simulink model "FullFilterTest"  (R2019b)
settings: Solver=FixedStepAuto  StartTime=0.0  StopTime=36  FixedStep=1  RelTol=1e-3
libraries: simulink x1
settings Model: Creator=pieterpinson  LastModifiedBy=pieterpinson

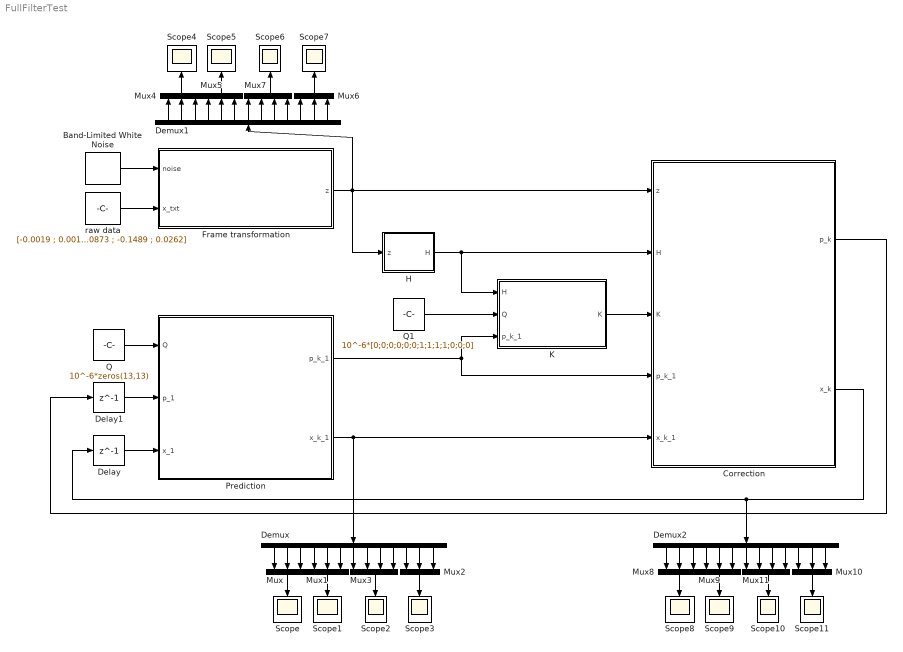
== system FullFilterTest ==
  Band-Limited White Noise : simulink/Sources/Band-Limited White Noise  Cov=[sin(sin(0.1))]  Ts=1  seed=[23341]
  Correction : MATLAB Function  TreatAsAtomicUnit=on
  Delay : Delay  DelayLength=1  InitialCondition=|
      | [-0.0019 ; 0.0017 ; 1.0891 ; 0 ; 0 ; 0 ; -0.7226 ; 0.6358 ; 0.1434 ; 0.2302
      | ; -0.0873 ; -0.1489 ; 0.0262]
  Delay1 : Delay  DelayLength=1  InitialCondition=ones(13,13)
  Demux : Demux  Outputs=13
  Demux1 : Demux  Outputs=13
  Demux2 : Demux  Outputs=13
  Frame transformation : MATLAB Function  TreatAsAtomicUnit=on
  H : MATLAB Function  TreatAsAtomicUnit=on
  K : MATLAB Function  TreatAsAtomicUnit=on
  Mux{,1..2,4..6,8..10} (9 alike) : Mux  Inputs=3
  Mux11 : Mux
  Mux3 : Mux
  Mux7 : Mux
  Prediction : MATLAB Function  TreatAsAtomicUnit=on
  Q : Constant  Value=10^-6*zeros(13,13)
  Q1 : Constant  Value=10^-6*[0;0;0;0;0;0;1;1;1;1;0;0;0]
  Scope{,1..11} (12 alike) : Scope
  raw data : Constant  Value=|
      | [-0.0019 ; 0.0017 ; 1.0891 ; 0 ; 0 ; 0 ; -0.7226 ; 0.6358 ; 0.1434 ; 0.2302
      | ; -0.0873 ; -0.1489 ; 0.0262]
  wires:
  Prediction/2(x_k_1) -> Demux/1, Correction/5(x_k_1)
  Mux3/1 -> Scope2/1
  Demux/13 -> Mux2/3
  Demux/12 -> Mux2/2
  Demux/11 -> Mux2/1
  Demux/10 -> Mux3/4
  Demux/9 -> Mux3/3
  Demux/8 -> Mux3/2
  Demux/7 -> Mux3/1
  Demux/6 -> Mux1/3
  Demux/5 -> Mux1/2
  Demux/4 -> Mux1/1
  Demux/3 -> Mux/3
  Demux/2 -> Mux/2
  Demux/1 -> Mux/1
  Mux1/1 -> Scope1/1
  Mux/1 -> Scope/1
  Delay/1 -> Prediction/3(x_1)
  Mux2/1 -> Scope3/1
  Q/1 -> Prediction/1(Q)
  Delay1/1 -> Prediction/2(p_1)
  raw data/1 -> Frame transformation/2(x_txt)
  Band-Limited White Noise/1 -> Frame transformation/1(noise)
  Mux6/1 -> Scope7/1
  Demux1/3 -> Mux4/3
  Demux1/10 -> Mux7/4
  Demux1/2 -> Mux4/2
  Demux1/1 -> Mux4/1
  Demux1/11 -> Mux6/1
  Mux4/1 -> Scope4/1
  Mux5/1 -> Scope5/1
  Mux7/1 -> Scope6/1
  Demux1/6 -> Mux5/3
  Demux1/9 -> Mux7/3
  Demux1/13 -> Mux6/3
  Demux1/12 -> Mux6/2
  Demux1/7 -> Mux7/1
  Frame transformation/1(z) -> H/1(z), Correction/1(z), Demux1/1
  Demux1/4 -> Mux5/1
  Demux1/5 -> Mux5/2
  Demux1/8 -> Mux7/2
  H/1(H) -> K/1(H), Correction/2(H)
  Correction/1(p_k) -> Delay1/1
  Correction/2(x_k) -> Demux2/1, Delay/1
  Mux10/1 -> Scope11/1
  Demux2/3 -> Mux8/3
  Demux2/10 -> Mux11/4
  Demux2/2 -> Mux8/2
  Demux2/1 -> Mux8/1
  Demux2/11 -> Mux10/1
  Mux8/1 -> Scope8/1
  Mux9/1 -> Scope9/1
  Mux11/1 -> Scope10/1
  Demux2/6 -> Mux9/3
  Demux2/9 -> Mux11/3
  Demux2/4 -> Mux9/1
  Demux2/13 -> Mux10/3
  Demux2/12 -> Mux10/2
  Demux2/7 -> Mux11/1
  Demux2/5 -> Mux9/2
  Demux2/8 -> Mux11/2
  Prediction/1(p_k_1) -> K/3(p_k_1), Correction/4(p_k_1)
  K/1(K) -> Correction/3(K)
  Q1/1 -> K/2(Q)

== matlab function FullFilterTest/Frame transformation ==
  data: noise input; x_txt input; z output
function z = PnPsolver(noise,x_txt)

%PnP solve magie
z = 1*x_txt + noise;

end

== matlab function FullFilterTest/Prediction ==
  data: Q input; p_1 input; p_k_1 output; x_k_1 output; x_1 input
function [p_k_1,x_k_1]= prediction(Q,p_1,x_1)

%orbital parameter
mu = 3.986*10^14;
R_earth = 6371000;
H_target = 773000;
a = R_earth + H_target;
n = sqrt(mu/(a^3));

%clohessy-wiltshire equations
dr = [4-3*cos(n) 0 0 sin(n)/n 2*(1-cos(n))/n 0 ; 6*(sin(n)-n) 1 0 2*(cos(n)-1)/n (4*sin(n)-3*n)/n 0 ; 0 0 cos(n) 0 0 sin(n)/n];
dv = [3*n*sin(n) 0 0 cos(n) 2*sin(n) 0 ; 6*n*(cos(n)-1) 0 0 -2*sin(n) 4*cos(n)-3 0 ; 0 0 -n*sin(n) 0 0 cos(n)];

%quaternion kinematic equation
dq = 0.5*[0 x_1(13) -x_1(12) x_1(11) ; -x_1(13) 0 x_1(11) x_1(12) ; x_1(12) -x_1(11) 0 x_1(13) ; -x_1(11) -x_1(12) -x_1(13) 0];

%state transition matrix
fi = [dr zeros(3,7) ; dv zeros(3,7) ; zeros(4,6) dq zeros(4,3) ; zeros(3,10) eye(3)];

%propogation step
x_k_1 = [0;0;0;0;0;0;x_1(7:10);0;0;0] + fi * x_1;
p_k_1 = fi * p_1 * fi.' + Q;

end


%dq1 = 0.5*[x_1(10) -x_1(9) x_1(8) x_1(7) ; x_1(9) x_1(10) -x_1(7) x_1(8) ; -x_1(8) x_1(7) x_1(10) x_1(9) ; -x_1(7) -x_1(8) -x_1(9) x_1(10)];
%fi(7,7) = x_1(7) + 0.5*(x_1(12)*x_1(8) - x_1(12)*x_1(9) + x_1(11)*x_1(10));
%fi(8,8) = x_1(8) + 0.5*(-x_1(13)*x_1(7) + x_1(11)*x_1(9) + x_1(12)*x_1(10));
%fi(9,9) = x_1(9) + 0.5*(x_1(12)*x_1(7) - x_1(11)*x_1(8) + x_1(13)*x_1(10));
%fi(10,10) = x_1(10) + 0.5*(-x_1(11)*x_1(7) - x_1(12)*x_1(8) - x_1(13)*x_1(9));

== matlab function FullFilterTest/Correction ==
  data: z input; p_k output; x_k output; H input; K input; p_k_1 input; x_k_1 input
function [p_k,x_k]= correction(z,H,K,p_k_1,x_k_1)

%correction step
x_k = x_k_1 + K.*(z - H.'*z);
p_k = (eye(13,13) - K*H)*p_k_1;

end

== matlab function FullFilterTest/H ==
  data: z input; H output
function H = jacobian(z)

%jacobian tranformation magic
H = z;

end

== matlab function FullFilterTest/K ==
  data: H input; Q input; K output; p_k_1 input
function K = kalmangain(H,Q,p_k_1)

%kalman gain calculation
K = p_k_1 * H.' * inv(H * p_k_1 * H.' + Q);

end
